simulink model "Control_try_final_2020b"  (R2020b)
settings: Solver=VariableStepAuto  StartTime=0.0  StopTime=inf  RelTol=1e-3
undefined symbols (not defined in the file or in its folder): DiscIntNeverNeededParam
libraries: mobileRoboticsLib x25
(part 1 of 7)
settings Model: Creator=its_ghani  LastModifiedBy=nitis
settings DebuggingCC: SFMachineParentedDataDiag=error  UnderSpecifiedDimensionMsg=warning

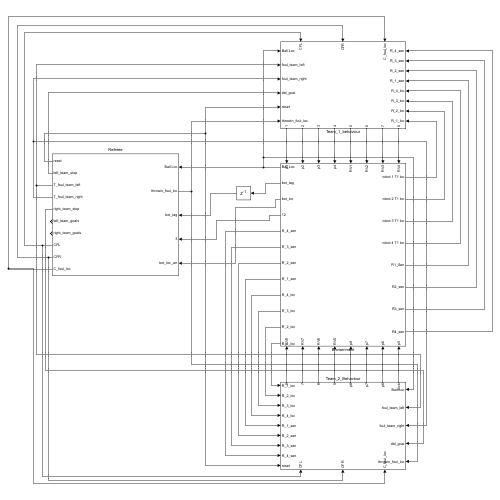
[thumbnail: Simulink's stored preview of the top-level diagram]
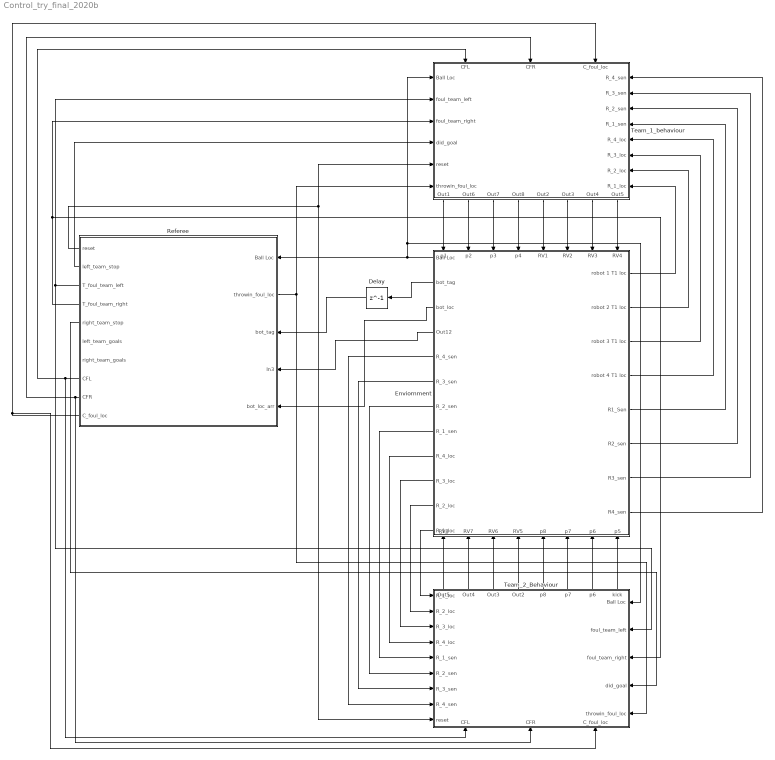
== system Control_try_final_2020b ==
  Delay : Delay  DelayLength=1
  Enviornment : Subsystem
      settings: PortSchema="{\"entries\":[{\"content\":{\"sides\":[{\"content\":{\"connectorIds\":[\"Out9\",\"Out10\",\"Out11\",\"Out12\",\"Out13\",\"Out14\",\"Out15\",\"Out16\",\"Out17\",\"Out18\",\"Out19\",\"Out20\"]},\"type\":\"ConnectorPlacement.EquallySpacedRectSide\",\"uuid\":\"bfc4f995-18bb-40a5-813e-439d500b4bf9\"},{\"content\":{\"connectorIds\":[\"Out1\",\"Out2\",\"Out3\",\"Out4\",\"Out5\",\"Out6\",\"Out7\",\"Out8\"],\"side\":\"RIGHT\"},\"type\":\"ConnectorPlacement.EquallySpacedRectSide\",\"uuid\":\"3fb6b8a6-16df-4a59-8ba5-6321e26d1fdd\"},{\"content\":{\"connectorIds\":[\"In1\",\"In2\",\"In3\",\"In4\",\"In5\",\"In6\",\"In7\",\"In8\"],\"side\":\"TOP\"},\"type\":\"ConnectorPlacement.EquallySpacedRectSide\",\"uuid\":\"a9e4cd1b-3afe-4395-99fa-15aef12a4070\"},{\"content\":{\"connectorIds\":[\"In9\",\"In10\",\"In11\",\"In12\",\"In13\",\"In14\",\"In15\",\"In16\"],\"side\":\"BOTTOM\"},\"type\":\"ConnectorPlacement.EquallySpacedRectSide\",\"uuid\":\"078de565-4bd1-4f1b-9c98-125152a73844\"}]},\"type\":\"ConnectorPlacement.EquallySpacedConnector\",\"uuid\":\"a6ca697e-fe67-43ac-b669-91f3e6c836c9\"}],\"packageUris\":[\"http://schema.mathworks.com/mf0/Connector/R2020b\"],\"version\":\"1.0\"}"
  Referee : Subsystem
      settings: PortSchema="{\"entries\":[{\"content\":{\"sides\":[{\"content\":{\"connectorIds\":[\"In1\",\"Out11\",\"In2\",\"In3\",\"In4\"]},\"type\":\"ConnectorPlacement.EquallySpacedRectSide\",\"uuid\":\"24b9e11e-cd74-4a0c-9d20-0512ace72e94\"},{\"content\":{\"connectorIds\":[\"Out1\",\"Out2\",\"Out3\",\"Out4\",\"Out5\",\"Out6\",\"Out7\",\"Out8\",\"Out9\",\"Out10\"],\"side\":\"RIGHT\"},\"type\":\"ConnectorPlacement.EquallySpacedRectSide\",\"uuid\":\"9dfe8633-4d3d-43ab-8a9b-a2838e7b041b\"},{\"content\":{\"connectorIds\":[],\"side\":\"TOP\"},\"type\":\"ConnectorPlacement.EquallySpacedRectSide\",\"uuid\":\"dd8f60d5-a719-4603-9445-e84921578fa6\"}]},\"type\":\"ConnectorPlacement.EquallySpacedConnector\",\"uuid\":\"54df3931-ee61-4f2f-89b6-33f93cd52d65\"}],\"packageUris\":[\"http://schema.mathworks.com/mf0/Connector/R2020b\"],\"version\":\"1.0\"}"
  Team_1_behaviour : Subsystem
      settings: PortSchema="{\"entries\":[{\"content\":{\"sides\":[{\"content\":{\"connectorIds\":[\"In1\",\"In2\",\"In3\",\"In4\",\"In5\",\"In6\"]},\"type\":\"ConnectorPlacement.EquallySpacedRectSide\",\"uuid\":\"3d238569-03e8-47ba-93af-d09e13fdb2d4\"},{\"content\":{\"connectorIds\":[\"In10\",\"In11\",\"In12\",\"In13\",\"In14\",\"In15\",\"In16\",\"In17\"],\"side\":\"RIGHT\"},\"type\":\"ConnectorPlacement.EquallySpacedRectSide\",\"uuid\":\"12d8afb4-4727-4f82-8566-507ab080c6de\"},{\"content\":{\"connectorIds\":[\"In7\",\"In8\",\"In9\"],\"side\":\"TOP\"},\"type\":\"ConnectorPlacement.EquallySpacedRectSide\",\"uuid\":\"c52fa7ec-51b7-43be-84ca-6ce417c012c7\"},{\"content\":{\"connectorIds\":[\"Out1\",\"Out2\",\"Out3\",\"Out4\",\"Out5\",\"Out6\",\"Out7\",\"Out8\"],\"side\":\"BOTTOM\"},\"type\":\"ConnectorPlacement.EquallySpacedRectSide\",\"uuid\":\"1ba4ac49-8e90-4b3f-8374-c14756940453\"}]},\"type\":\"ConnectorPlacement.EquallySpacedConnector\",\"uuid\":\"883bb5df-d6b2-498f-94a4-3b94e28c6a8f\"}],\"packageUris\":[\"http://schema.mathworks.com/mf0/Connector/R2020b\"],\"version\":\"1.0\"}"
  Team_2_Behaviour : Subsystem
      settings: PortSchema="{\"entries\":[{\"content\":{\"sides\":[{\"content\":{\"connectorIds\":[\"In1\",\"In2\",\"In3\",\"In4\",\"In5\"]},\"type\":\"ConnectorPlacement.EquallySpacedRectSide\",\"uuid\":\"3d238569-03e8-47ba-93af-d09e13fdb2d4\"},{\"content\":{\"connectorIds\":[\"In9\",\"In10\",\"In11\",\"In12\",\"In13\",\"In14\",\"In15\",\"In16\",\"In17\"],\"side\":\"RIGHT\"},\"type\":\"ConnectorPlacement.EquallySpacedRectSide\",\"uuid\":\"12d8afb4-4727-4f82-8566-507ab080c6de\"},{\"content\":{\"connectorIds\":[\"In6\",\"In7\",\"In8\"],\"side\":\"TOP\"},\"type\":\"ConnectorPlacement.EquallySpacedRectSide\",\"uuid\":\"c52fa7ec-51b7-43be-84ca-6ce417c012c7\"},{\"content\":{\"connectorIds\":[\"Out1\",\"Out2\",\"Out3\",\"Out4\",\"Out5\",\"Out6\",\"Out7\",\"Out8\"],\"side\":\"BOTTOM\"},\"type\":\"ConnectorPlacement.EquallySpacedRectSide\",\"uuid\":\"1ba4ac49-8e90-4b3f-8374-c14756940453\"}]},\"type\":\"ConnectorPlacement.EquallySpacedConnector\",\"uuid\":\"883bb5df-d6b2-498f-94a4-3b94e28c6a8f\"}],\"packageUris\":[\"http://schema.mathworks.com/mf0/Connector/R2020b\"],\"version\":\"1.0\"}"
  wires:
  Enviornment/9(Ball Loc) -> Team_1_behaviour/1(Ball Loc), Team_2_Behaviour/5(Ball Loc), Referee/1(Ball Loc)
  Team_1_behaviour/5(Out2) -> Enviornment/5(RV1)
  Team_1_behaviour/6(Out3) -> Enviornment/6(RV2)
  Team_1_behaviour/7(Out4) -> Enviornment/7(RV3)
  Team_1_behaviour/8(Out5) -> Enviornment/8(RV4)
  Enviornment/1(robot 1 T1 loc) -> Team_1_behaviour/17(R_1_loc)
  Enviornment/2(robot 2 T1 loc) -> Team_1_behaviour/16(R_2_loc)
  Enviornment/3(robot 3 T1 loc) -> Team_1_behaviour/15(R_3_loc)
  Enviornment/4(robot 4 T1 loc) -> Team_1_behaviour/14(R_4_loc)
  Enviornment/5(R1_Sen) -> Team_1_behaviour/13(R_1_sen)
  Enviornment/6(R2_sen) -> Team_1_behaviour/12(R_2_sen)
  Enviornment/7(R3_sen) -> Team_1_behaviour/11(R_3_sen)
  Enviornment/8(R4_sen) -> Team_1_behaviour/10(R_4_sen)
  Team_1_behaviour/2(Out6) -> Enviornment/2(p2)
  Team_1_behaviour/3(Out7) -> Enviornment/3(p3)
  Team_1_behaviour/4(Out8) -> Enviornment/4(p4)
  Enviornment/10(bot_tag) -> Delay/1
  Enviornment/11(bot_loc) -> Referee/4(bot_loc_arr)
  Team_2_Behaviour/1(kick) -> Enviornment/16(p5)
  Team_2_Behaviour/2(p6) -> Enviornment/15(p6)
  Team_2_Behaviour/3(p7) -> Enviornment/14(p7)
  Team_2_Behaviour/4(p8) -> Enviornment/13(p8)
  Team_2_Behaviour/5(Out2) -> Enviornment/12(RV5)
  Team_2_Behaviour/6(Out3) -> Enviornment/11(RV6)
  Team_2_Behaviour/7(Out4) -> Enviornment/10(RV7)
  Team_2_Behaviour/8(Out5) -> Enviornment/9(RV8)
  Enviornment/20(R_1_loc) -> Team_2_Behaviour/17(R_1_loc)
  Enviornment/19(R_2_loc) -> Team_2_Behaviour/16(R_2_loc)
  Enviornment/18(R_3_loc) -> Team_2_Behaviour/15(R_3_loc)
  Enviornment/17(R_4_loc) -> Team_2_Behaviour/14(R_4_loc)
  Enviornment/16(R_1_sen) -> Team_2_Behaviour/13(R_1_sen)
  Enviornment/15(R_2_sen) -> Team_2_Behaviour/12(R_2_sen)
  Enviornment/14(R_3_sen) -> Team_2_Behaviour/11(R_3_sen)
  Enviornment/13(R_4_sen) -> Team_2_Behaviour/10(R_4_sen)
  Team_1_behaviour/1(Out1) -> Enviornment/1(p1)
  Referee/1(reset) -> Team_1_behaviour/5(reset), Team_2_Behaviour/9(reset)
  Referee/2(left_team_stop) -> Team_1_behaviour/4(did_goal)
  Referee/5(right_team_stop) -> Team_2_Behaviour/2(did_goal)
  Referee/3(T_foul_team_left) -> Team_2_Behaviour/4(foul_team_left), Team_1_behaviour/2(foul_team_left)
  Referee/4(T_foul_team_right) -> Team_2_Behaviour/3(foul_team_right), Team_1_behaviour/3(foul_team_right)
  Referee/11(throwin_foul_loc) -> Team_2_Behaviour/1(throwin_foul_loc), Team_1_behaviour/6(throwin_foul_loc)
  Delay/1 -> Referee/2(bot_tag)
  Referee/8(CFL) -> Team_1_behaviour/7(CFL), Team_2_Behaviour/8(CFL)
  Referee/9(CFR) -> Team_1_behaviour/8(CFR), Team_2_Behaviour/7(CFR)
  Referee/10(C_foul_loc) -> Team_2_Behaviour/6(C_foul_loc), Team_1_behaviour/9(C_foul_loc)
  Enviornment/12(Out12) -> Referee/3(In3)

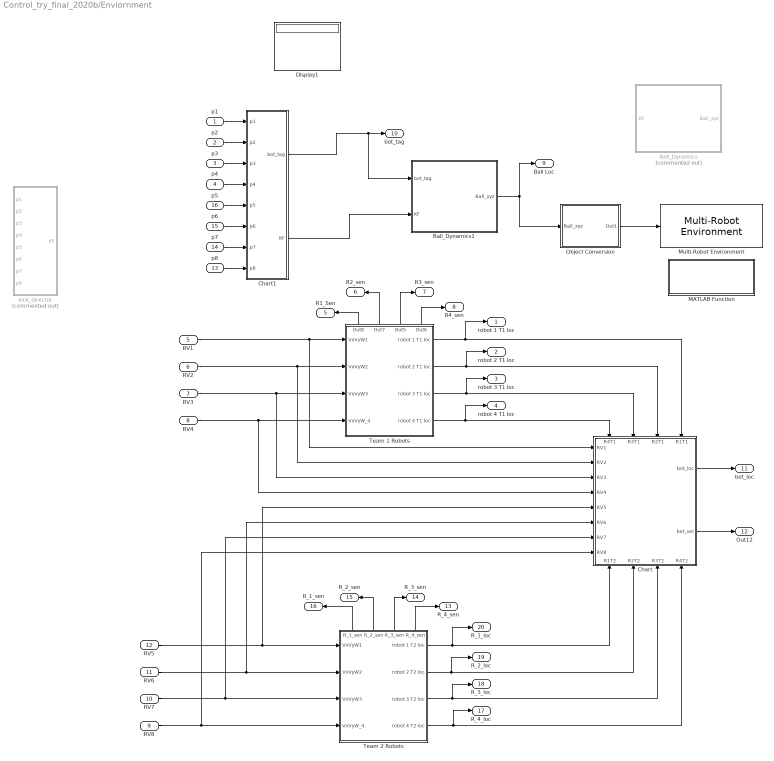
== system Control_try_final_2020b/Enviornment ==
  p1 : Inport  PortDimensions=4
  p2 : Inport  Port=2  PortDimensions=4
  p3 : Inport  Port=3  PortDimensions=4
  p4 : Inport  Port=4  PortDimensions=4
  RV1 : Inport  Port=5
  RV2 : Inport  Port=6
  RV3 : Inport  Port=7
  RV4 : Inport  Port=8
  RV8 : Inport  Port=9
  RV7 : Inport  Port=10
  RV6 : Inport  Port=11
  RV5 : Inport  Port=12
  p8 : Inport  Port=13  PortDimensions=4
  p7 : Inport  Port=14  PortDimensions=4
  p6 : Inport  Port=15  PortDimensions=4
  p5 : Inport  Port=16  PortDimensions=4
  "\tTeam 1 Robots" : Subsystem
      settings: PortSchema="{\"entries\":[{\"content\":{\"sides\":[{\"content\":{\"connectorIds\":[\"In1\",\"In2\",\"In3\",\"In4\"]},\"type\":\"ConnectorPlacement.EquallySpacedRectSide\",\"uuid\":\"e759642f-fbca-4f1e-b212-daca2c4962f8\"},{\"content\":{\"connectorIds\":[\"Out1\",\"Out2\",\"Out3\",\"Out4\"],\"side\":\"RIGHT\"},\"type\":\"ConnectorPlacement.EquallySpacedRectSide\",\"uuid\":\"6e1699fa-b246-4758-836f-1d4c98857b70\"},{\"content\":{\"connectorIds\":[\"Out5\",\"Out6\",\"Out7\",\"Out8\"],\"side\":\"TOP\"},\"type\":\"ConnectorPlacement.EquallySpacedRectSide\",\"uuid\":\"c1cf0a96-808a-4241-9d01-181cc4ce2a4d\"},{\"content\":{\"connectorIds\":[],\"side\":\"BOTTOM\"},\"type\":\"ConnectorPlacement.EquallySpacedRectSide\",\"uuid\":\"1a7f648f-16d5-4a09-b479-d6590fa53252\"}]},\"type\":\"ConnectorPlacement.EquallySpacedConnector\",\"uuid\":\"5972ed04-ecdd-4117-bf5d-456318b5c4b8\"}],\"packageUris\":[\"http://schema.mathworks.com/mf0/Connector/R2020b\"],\"version\":\"1.0\"}"
  "\tTeam 2 Robots" : Subsystem
      settings: PortSchema="{\"entries\":[{\"content\":{\"sides\":[{\"content\":{\"connectorIds\":[\"In1\",\"In2\",\"In3\",\"In4\"]},\"type\":\"ConnectorPlacement.EquallySpacedRectSide\",\"uuid\":\"e759642f-fbca-4f1e-b212-daca2c4962f8\"},{\"content\":{\"connectorIds\":[\"Out1\",\"Out2\",\"Out3\",\"Out4\"],\"side\":\"RIGHT\"},\"type\":\"ConnectorPlacement.EquallySpacedRectSide\",\"uuid\":\"6e1699fa-b246-4758-836f-1d4c98857b70\"},{\"content\":{\"connectorIds\":[\"Out5\",\"Out6\",\"Out7\",\"Out8\"],\"side\":\"TOP\"},\"type\":\"ConnectorPlacement.EquallySpacedRectSide\",\"uuid\":\"c1cf0a96-808a-4241-9d01-181cc4ce2a4d\"},{\"content\":{\"connectorIds\":[],\"side\":\"BOTTOM\"},\"type\":\"ConnectorPlacement.EquallySpacedRectSide\",\"uuid\":\"1a7f648f-16d5-4a09-b479-d6590fa53252\"}]},\"type\":\"ConnectorPlacement.EquallySpacedConnector\",\"uuid\":\"5972ed04-ecdd-4117-bf5d-456318b5c4b8\"}],\"packageUris\":[\"http://schema.mathworks.com/mf0/Connector/R2020b\"],\"version\":\"1.0\"}"
  Ball_Dynamics : Subsystem  Commented=on
  Ball_Dynamics1 : Subsystem
  Chart : Stateflow chart  TreatAsAtomicUnit=on
      settings: PortSchema="{\"entries\":[{\"content\":{\"sides\":[{\"content\":{\"connectorIds\":[\"In1\",\"In2\",\"In3\",\"In4\",\"In6\",\"In7\",\"In5\",\"In8\"]},\"type\":\"ConnectorPlacement.EquallySpacedRectSide\",\"uuid\":\"f94597f5-b931-46ba-a6a2-82ef940fcb13\"},{\"content\":{\"connectorIds\":[\"Out1\",\"Out2\"],\"side\":\"RIGHT\"},\"type\":\"ConnectorPlacement.EquallySpacedRectSide\",\"uuid\":\"0de80a09-1ed4-4b2b-aafe-6337a06ba998\"},{\"content\":{\"connectorIds\":[\"In13\",\"In14\",\"In15\",\"In16\"],\"side\":\"TOP\"},\"type\":\"ConnectorPlacement.EquallySpacedRectSide\",\"uuid\":\"f3cbd75f-0570-4224-b4a7-f582d3326f83\"},{\"content\":{\"connectorIds\":[\"In9\",\"In10\",\"In11\",\"In12\"],\"side\":\"BOTTOM\"},\"type\":\"ConnectorPlacement.EquallySpacedRectSide\",\"uuid\":\"407d67c2-1282-447f-b8c3-2ff3cae03a1f\"}]},\"type\":\"ConnectorPlacement.EquallySpacedConnector\",\"uuid\":\"17e3c346-79d8-441f-9c0c-3b96471ef7ab\"}],\"packageUris\":[\"http://schema.mathworks.com/mf0/Connector/R2020b\"],\"version\":\"1.0\"}"
  Chart1 : Stateflow chart  TreatAsAtomicUnit=on
  Display1 : Display
  MATLAB Function : MATLAB Function  TreatAsAtomicUnit=on
  Multi-Robot Environment : mobileRoboticsLib/Environments/Multi-Robot Environment  numRobots=8  showWaypoints=off  showObjects=on  objectColors=[1 0 0;0 1 0;0 0 1]  objectMarkers='c'  showRobotIds=on  plotSensorLines=on
      settings: SourceProductName=Mobile Robotics Simulation Toolbox
  Object Conversion : Subsystem
  kick_director : Subsystem  Commented=on
  robot 1 T1 loc : Outport
  robot 2 T1 loc : Outport  Port=2
  robot 3 T1 loc : Outport  Port=3
  robot 4 T1 loc : Outport  Port=4
  R1_Sen : Outport  Port=5
  R2_sen : Outport  Port=6
  R3_sen : Outport  Port=7
  R4_sen : Outport  Port=8
  Ball Loc : Outport  Port=9
  bot_tag : Outport  Port=10
  bot_loc : Outport  Port=11
  Out12 : Outport  Port=12
  R_4_sen : Outport  Port=13
  R_3_sen : Outport  Port=14
  R_2_sen : Outport  Port=15
  R_1_sen : Outport  Port=16
  R_4_loc : Outport  Port=17
  R_3_loc : Outport  Port=18
  R_2_loc : Outport  Port=19
  R_1_loc : Outport  Port=20
  wires:
  "\tTeam 1 Robots"/1(robot 1 T1 loc) -> robot 1 T1 loc/1, Chart/16(R1T1)
  Object Conversion/1(Out1) -> Multi-Robot Environment/1
  "\tTeam 1 Robots"/2(robot 2 T1 loc) -> robot 2 T1 loc/1, Chart/15(R2T1)
  "\tTeam 1 Robots"/3(robot 3 T1 loc) -> robot 3 T1 loc/1, Chart/14(R3T1)
  "\tTeam 1 Robots"/4(robot 4 T1 loc) -> robot 4 T1 loc/1, Chart/13(R4T1)
  RV1/1 -> Chart/1(RV1), "\tTeam 1 Robots"/1(VxVyW1)
  "\tTeam 1 Robots"/5(Out8) -> R1_Sen/1
  "\tTeam 1 Robots"/6(Out7) -> R2_sen/1
  "\tTeam 1 Robots"/7(Out5) -> R3_sen/1
  "\tTeam 1 Robots"/8(Out6) -> R4_sen/1
  "\tTeam 2 Robots"/4(robot 4 T2 loc) -> R_4_loc/1, Chart/12(R4T2)
  "\tTeam 2 Robots"/1(robot 1 T2 loc) -> R_1_loc/1, Chart/9(R1T2)
  "\tTeam 2 Robots"/2(robot 2 T2 loc) -> R_2_loc/1, Chart/10(R2T2)
  "\tTeam 2 Robots"/3(robot 3 T2 loc) -> R_3_loc/1, Chart/11(R3T2)
  Chart/1(bot_loc) -> bot_loc/1
  Ball_Dynamics1/1(Ball_xyz) -> Ball Loc/1, Object Conversion/1(Ball_xyz)
  RV5/1 -> Chart/6(RV5), "\tTeam 2 Robots"/1(VxVyW1)
  "\tTeam 2 Robots"/6(R_2_sen) -> R_2_sen/1
  "\tTeam 2 Robots"/7(R_3_sen) -> R_3_sen/1
  "\tTeam 2 Robots"/5(R_1_sen) -> R_1_sen/1
  "\tTeam 2 Robots"/8(R_4_sen) -> R_4_sen/1
  p1/1 -> Chart1/1(p1)
  p2/1 -> Chart1/2(p2)
  p3/1 -> Chart1/3(p3)
  p4/1 -> Chart1/4(p4)
  p5/1 -> Chart1/5(p5)
  p6/1 -> Chart1/6(p6)
  p7/1 -> Chart1/7(p7)
  p8/1 -> Chart1/8(p8)
  Chart1/2(KF) -> Ball_Dynamics1/2(KF)
  Chart1/1(bot_tag) -> Ball_Dynamics1/1(bot_tag), bot_tag/1
  RV8/1 -> Chart/8(RV8), "\tTeam 2 Robots"/4(VxVyW_4)
  RV2/1 -> Chart/2(RV2), "\tTeam 1 Robots"/2(VxVyW2)
  RV3/1 -> Chart/3(RV3), "\tTeam 1 Robots"/3(VxVyW3)
  RV4/1 -> Chart/4(RV4), "\tTeam 1 Robots"/4(VxVyW_4)
  RV6/1 -> Chart/7(RV6), "\tTeam 2 Robots"/2(VxVyW2)
  RV7/1 -> Chart/5(RV7), "\tTeam 2 Robots"/3(VxVyW3)
  Chart/2(bot_vel) -> Out12/1

== system Control_try_final_2020b/Referee ==
  Ball Loc : Inport
  bot_tag : Inport  Port=2
  In3 : Inport  Port=3
  bot_loc_arr : Inport  Port=4
  Chart : Stateflow chart  TreatAsAtomicUnit=on
  Corner : Stateflow chart  TreatAsAtomicUnit=on
  Demux : Demux  Outputs=3
  GOAL : Stateflow chart  TreatAsAtomicUnit=on
      settings: PortSchema="{\"entries\":[{\"content\":{\"sides\":[{\"content\":{\"connectorIds\":[\"In1\",\"In2\",\"In3\"]},\"type\":\"ConnectorPlacement.EquallySpacedRectSide\",\"uuid\":\"4d055f86-b6e4-40f8-8e5a-f88426a8f4c4\"},{\"content\":{\"connectorIds\":[\"Out1\",\"Out5\",\"Out3\",\"Out4\",\"Out2\"],\"side\":\"RIGHT\"},\"type\":\"ConnectorPlacement.EquallySpacedRectSide\",\"uuid\":\"6dafae19-6ec2-41d7-a60c-cff09e299cdb\"},{\"content\":{\"connectorIds\":[],\"side\":\"TOP\"},\"type\":\"ConnectorPlacement.EquallySpacedRectSide\",\"uuid\":\"9f5e82fb-41f6-4c76-b3de-1e77cfc54a18\"}]},\"type\":\"ConnectorPlacement.EquallySpacedConnector\",\"uuid\":\"d854df09-5db2-4850-aa8e-94906c2af310\"}],\"packageUris\":[\"http://schema.mathworks.com/mf0/Connector/R2020b\"],\"version\":\"1.0\"}"
  Throwing : Stateflow chart  TreatAsAtomicUnit=on
  reset : Outport
  left_team_stop : Outport  Port=2
  T_foul_team_left : Outport  Port=3
  T_foul_team_right : Outport  Port=4
  right_team_stop : Outport  Port=5
  left_team_goals : Outport  Port=6
  right_team_goals : Outport  Port=7
  CFL : Outport  Port=8
  CFR : Outport  Port=9
  C_foul_loc : Outport  Port=10
  throwin_foul_loc : Outport  Port=11
  wires:
  Ball Loc/1 -> Demux/1
  Demux/1 -> GOAL/1(X), Throwing/1(X), Corner/2(X)
  Demux/2 -> GOAL/2(Y), Throwing/3(Y), Corner/3(Y)
  Demux/3 -> GOAL/3(Z)
  GOAL/1(left_team_goal) -> left_team_goals/1
  GOAL/5(right_team_goal) -> right_team_goals/1
  GOAL/2(reset) -> reset/1
  bot_tag/1 -> Corner/1(ball_tag), Throwing/2(bot_tag)
  bot_loc_arr/1 -> Chart/2(bot_loc_arr)
  GOAL/4(right_team_stop) -> right_team_stop/1
  GOAL/3(left_team_stop) -> left_team_stop/1
  Throwing/2(foul_team_left) -> T_foul_team_left/1
  Throwing/1(foul_team_right) -> T_foul_team_right/1
  Throwing/3(throwin_foul_loc) -> throwin_foul_loc/1
  Corner/3(C_foul_loc) -> C_foul_loc/1
  Corner/2(CFL) -> CFL/1
  Corner/1(CFR) -> CFR/1
  In3/1 -> Chart/1(bot_vel)

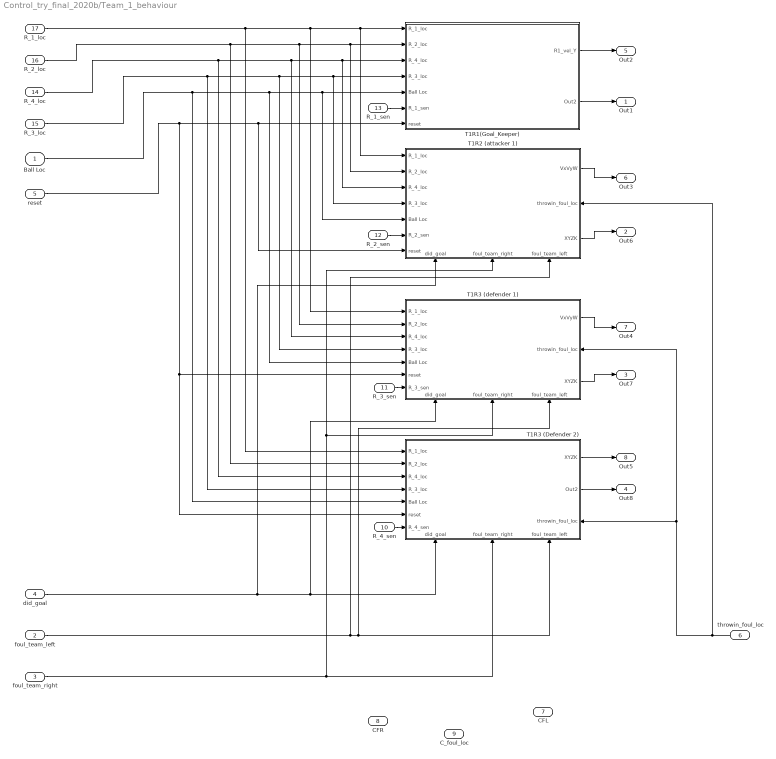
== system Control_try_final_2020b/Team_1_behaviour ==
  Ball Loc : Inport
  foul_team_left : Inport  Port=2
  foul_team_right : Inport  Port=3
  did_goal : Inport  Port=4
  reset : Inport  Port=5
  throwin_foul_loc : Inport  Port=6
  CFL : Inport  Port=7
  CFR : Inport  Port=8
  C_foul_loc : Inport  Port=9
  R_4_sen : Inport  Port=10
  R_3_sen : Inport  Port=11
  R_2_sen : Inport  Port=12
  R_1_sen : Inport  Port=13
  R_4_loc : Inport  Port=14
  R_3_loc : Inport  Port=15
  R_2_loc : Inport  Port=16
  R_1_loc : Inport  Port=17
  T1R1(Goal_Keeper) : Subsystem
  T1R2 (attacker 1) : Subsystem
      settings: PortSchema="{\"entries\":[{\"content\":{\"sides\":[{\"content\":{\"connectorIds\":[\"In1\",\"In2\",\"In3\",\"In4\",\"In5\",\"In6\",\"In7\"]},\"type\":\"ConnectorPlacement.EquallySpacedRectSide\",\"uuid\":\"970e53f5-0a77-471a-b839-4d72993ac113\"},{\"content\":{\"connectorIds\":[\"Out1\",\"In11\",\"Out2\"],\"side\":\"RIGHT\"},\"type\":\"ConnectorPlacement.EquallySpacedRectSide\",\"uuid\":\"b4f21133-1799-4814-963e-0f46ba79bd15\"},{\"content\":{\"connectorIds\":[],\"side\":\"TOP\"},\"type\":\"ConnectorPlacement.EquallySpacedRectSide\",\"uuid\":\"b11bbb03-05f4-411e-9610-26b6f9bf001d\"},{\"content\":{\"connectorIds\":[\"In8\",\"In9\",\"In10\"],\"side\":\"BOTTOM\"},\"type\":\"ConnectorPlacement.EquallySpacedRectSide\",\"uuid\":\"303a1a36-f5d7-4d15-b6f4-55568a48a6c3\"}]},\"type\":\"ConnectorPlacement.EquallySpacedConnector\",\"uuid\":\"9d40740d-7bec-4cd7-8121-739ec5dca381\"}],\"packageUris\":[\"http://schema.mathworks.com/mf0/Connector/R2020b\"],\"version\":\"1.0\"}"
  T1R3 (Defender 2) : Subsystem
      settings: PortSchema="{\"entries\":[{\"content\":{\"sides\":[{\"content\":{\"connectorIds\":[\"In1\",\"In2\",\"In3\",\"In4\",\"In5\",\"In6\",\"In7\"]},\"type\":\"ConnectorPlacement.EquallySpacedRectSide\",\"uuid\":\"970e53f5-0a77-471a-b839-4d72993ac113\"},{\"content\":{\"connectorIds\":[\"Out1\",\"Out2\",\"In11\"],\"side\":\"RIGHT\"},\"type\":\"ConnectorPlacement.EquallySpacedRectSide\",\"uuid\":\"b4f21133-1799-4814-963e-0f46ba79bd15\"},{\"content\":{\"connectorIds\":[],\"side\":\"TOP\"},\"type\":\"ConnectorPlacement.EquallySpacedRectSide\",\"uuid\":\"b11bbb03-05f4-411e-9610-26b6f9bf001d\"},{\"content\":{\"connectorIds\":[\"In8\",\"In9\",\"In10\"],\"side\":\"BOTTOM\"},\"type\":\"ConnectorPlacement.EquallySpacedRectSide\",\"uuid\":\"1ea9a003-1cbb-4940-9cbf-9a8dc4be1575\"}]},\"type\":\"ConnectorPlacement.EquallySpacedConnector\",\"uuid\":\"9d40740d-7bec-4cd7-8121-739ec5dca381\"}],\"packageUris\":[\"http://schema.mathworks.com/mf0/Connector/R2020b\"],\"version\":\"1.0\"}"
  T1R3 (defender 1) : Subsystem
      settings: PortSchema="{\"entries\":[{\"content\":{\"sides\":[{\"content\":{\"connectorIds\":[\"In1\",\"In2\",\"In3\",\"In4\",\"In5\",\"In6\",\"In7\"]},\"type\":\"ConnectorPlacement.EquallySpacedRectSide\",\"uuid\":\"970e53f5-0a77-471a-b839-4d72993ac113\"},{\"content\":{\"connectorIds\":[\"Out1\",\"In11\",\"Out2\"],\"side\":\"RIGHT\"},\"type\":\"ConnectorPlacement.EquallySpacedRectSide\",\"uuid\":\"b4f21133-1799-4814-963e-0f46ba79bd15\"},{\"content\":{\"connectorIds\":[],\"side\":\"TOP\"},\"type\":\"ConnectorPlacement.EquallySpacedRectSide\",\"uuid\":\"b11bbb03-05f4-411e-9610-26b6f9bf001d\"},{\"content\":{\"connectorIds\":[\"In8\",\"In9\",\"In10\"],\"side\":\"BOTTOM\"},\"type\":\"ConnectorPlacement.EquallySpacedRectSide\",\"uuid\":\"9d6502f6-0cb3-4e7b-b72a-712aec65b358\"}]},\"type\":\"ConnectorPlacement.EquallySpacedConnector\",\"uuid\":\"9d40740d-7bec-4cd7-8121-739ec5dca381\"}],\"packageUris\":[\"http://schema.mathworks.com/mf0/Connector/R2020b\"],\"version\":\"1.0\"}"
  Out1 : Outport
  Out6 : Outport  Port=2
  Out7 : Outport  Port=3
  Out8 : Outport  Port=4
  Out2 : Outport  Port=5
  Out3 : Outport  Port=6
  Out4 : Outport  Port=7
  Out5 : Outport  Port=8
  wires:
  T1R1(Goal_Keeper)/1(R1_vel_Y) -> Out2/1
  R_1_sen/1 -> T1R1(Goal_Keeper)/6(R_1_sen)
  R_1_loc/1 -> T1R3 (Defender 2)/1(R_1_loc), T1R3 (defender 1)/1(R_1_loc), T1R1(Goal_Keeper)/1(R_1_loc), T1R2 (attacker 1)/1(R_1_loc)
  R_2_loc/1 -> T1R3 (Defender 2)/2(R_2_loc), T1R3 (defender 1)/2(R_2_loc), T1R1(Goal_Keeper)/2(R_2_loc), T1R2 (attacker 1)/2(R_2_loc)
  R_4_loc/1 -> T1R3 (Defender 2)/3(R_4_loc), T1R3 (defender 1)/3(R_4_loc), T1R1(Goal_Keeper)/3(R_4_loc), T1R2 (attacker 1)/3(R_4_loc)
  R_3_loc/1 -> T1R3 (Defender 2)/4(R_3_loc), T1R3 (defender 1)/4(R_3_loc), T1R1(Goal_Keeper)/4(R_3_loc), T1R2 (attacker 1)/4(R_3_loc)
  Ball Loc/1 -> T1R3 (Defender 2)/5(Ball Loc), T1R3 (defender 1)/5(Ball Loc), T1R1(Goal_Keeper)/5(Ball Loc), T1R2 (attacker 1)/5(Ball Loc)
  R_2_sen/1 -> T1R2 (attacker 1)/6(R_2_sen)
  R_3_sen/1 -> T1R3 (defender 1)/7(R_3_sen)
  R_4_sen/1 -> T1R3 (Defender 2)/7(R_4_sen)
  T1R2 (attacker 1)/1(VxVyW) -> Out3/1
  T1R3 (defender 1)/1(VxVyW) -> Out4/1
  T1R3 (Defender 2)/1(XYZK) -> Out5/1
  T1R2 (attacker 1)/2(XYZK) -> Out6/1
  T1R3 (defender 1)/2(XYZK) -> Out7/1
  T1R3 (Defender 2)/2(Out2) -> Out8/1
  T1R1(Goal_Keeper)/2(Out2) -> Out1/1
  reset/1 -> T1R3 (defender 1)/6(reset), T1R3 (Defender 2)/6(reset), T1R1(Goal_Keeper)/7(reset), T1R2 (attacker 1)/7(reset)
  did_goal/1 -> T1R3 (Defender 2)/8(did_goal), T1R3 (defender 1)/8(did_goal), T1R2 (attacker 1)/8(did_goal)
  foul_team_left/1 -> T1R2 (attacker 1)/10(foul_team_left), T1R3 (defender 1)/10(foul_team_left), T1R3 (Defender 2)/10(foul_team_left)
  throwin_foul_loc/1 -> T1R2 (attacker 1)/11(throwin_foul_loc), T1R3 (defender 1)/11(throwin_foul_loc), T1R3 (Defender 2)/11(throwin_foul_loc)
  foul_team_right/1 -> T1R3 (defender 1)/9(foul_team_right), T1R2 (attacker 1)/9(foul_team_right), T1R3 (Defender 2)/9(foul_team_right)

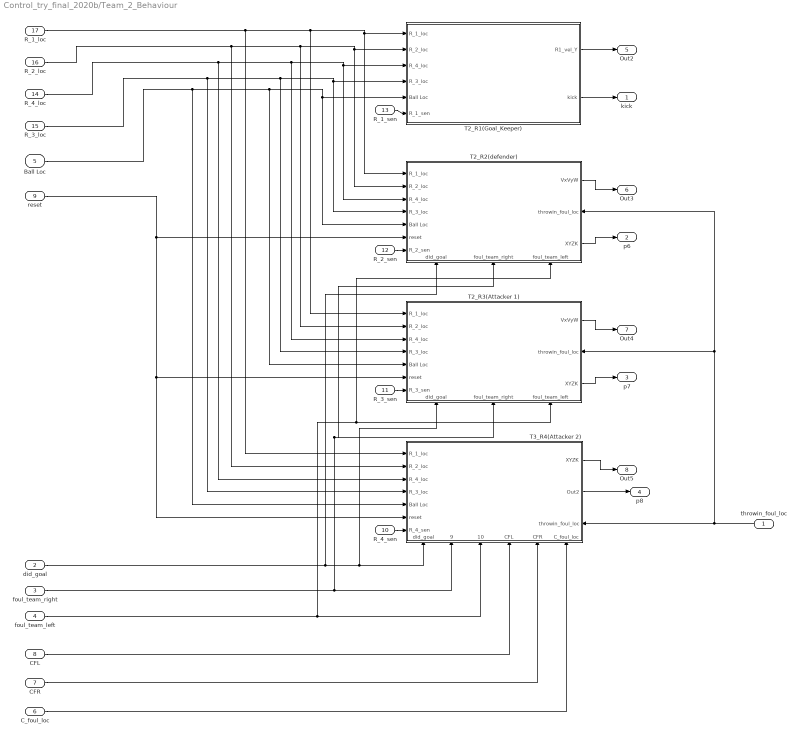
== system Control_try_final_2020b/Team_2_Behaviour ==
  throwin_foul_loc : Inport
  did_goal : Inport  Port=2
  foul_team_right : Inport  Port=3
  foul_team_left : Inport  Port=4
  Ball Loc : Inport  Port=5
  C_foul_loc : Inport  Port=6
  CFR : Inport  Port=7
  CFL : Inport  Port=8
  reset : Inport  Port=9
  R_4_sen : Inport  Port=10
  R_3_sen : Inport  Port=11
  R_2_sen : Inport  Port=12
  R_1_sen : Inport  Port=13
  R_4_loc : Inport  Port=14
  R_3_loc : Inport  Port=15
  R_2_loc : Inport  Port=16
  R_1_loc : Inport  Port=17
  T2_R1(Goal_Keeper) : Subsystem
  T2_R2(defender) : Subsystem
      settings: PortSchema="{\"entries\":[{\"content\":{\"sides\":[{\"content\":{\"connectorIds\":[\"In1\",\"In2\",\"In3\",\"In4\",\"In5\",\"In6\",\"In7\"]},\"type\":\"ConnectorPlacement.EquallySpacedRectSide\",\"uuid\":\"970e53f5-0a77-471a-b839-4d72993ac113\"},{\"content\":{\"connectorIds\":[\"Out1\",\"In11\",\"Out2\"],\"side\":\"RIGHT\"},\"type\":\"ConnectorPlacement.EquallySpacedRectSide\",\"uuid\":\"b4f21133-1799-4814-963e-0f46ba79bd15\"},{\"content\":{\"connectorIds\":[],\"side\":\"TOP\"},\"type\":\"ConnectorPlacement.EquallySpacedRectSide\",\"uuid\":\"b11bbb03-05f4-411e-9610-26b6f9bf001d\"},{\"content\":{\"connectorIds\":[\"In8\",\"In9\",\"In10\"],\"side\":\"BOTTOM\"},\"type\":\"ConnectorPlacement.EquallySpacedRectSide\",\"uuid\":\"e3d04837-b11c-4a80-91fc-07d9315080e1\"}]},\"type\":\"ConnectorPlacement.EquallySpacedConnector\",\"uuid\":\"9d40740d-7bec-4cd7-8121-739ec5dca381\"}],\"packageUris\":[\"http://schema.mathworks.com/mf0/Connector/R2020b\"],\"version\":\"1.0\"}"
  T2_R3(Attacker 1) : Subsystem
      settings: PortSchema="{\"entries\":[{\"content\":{\"sides\":[{\"content\":{\"connectorIds\":[\"In1\",\"In2\",\"In3\",\"In4\",\"In5\",\"In6\",\"In7\"]},\"type\":\"ConnectorPlacement.EquallySpacedRectSide\",\"uuid\":\"970e53f5-0a77-471a-b839-4d72993ac113\"},{\"content\":{\"connectorIds\":[\"Out1\",\"In11\",\"Out2\"],\"side\":\"RIGHT\"},\"type\":\"ConnectorPlacement.EquallySpacedRectSide\",\"uuid\":\"b4f21133-1799-4814-963e-0f46ba79bd15\"},{\"content\":{\"connectorIds\":[],\"side\":\"TOP\"},\"type\":\"ConnectorPlacement.EquallySpacedRectSide\",\"uuid\":\"b11bbb03-05f4-411e-9610-26b6f9bf001d\"},{\"content\":{\"connectorIds\":[\"In8\",\"In9\",\"In10\"],\"side\":\"BOTTOM\"},\"type\":\"ConnectorPlacement.EquallySpacedRectSide\",\"uuid\":\"51c3f414-bb29-49ed-bca1-9e09266b77a9\"}]},\"type\":\"ConnectorPlacement.EquallySpacedConnector\",\"uuid\":\"9d40740d-7bec-4cd7-8121-739ec5dca381\"}],\"packageUris\":[\"http://schema.mathworks.com/mf0/Connector/R2020b\"],\"version\":\"1.0\"}"
  T3_R4(Attacker 2) : Subsystem
      settings: PortSchema="{\"entries\":[{\"content\":{\"sides\":[{\"content\":{\"connectorIds\":[\"In1\",\"In2\",\"In3\",\"In4\",\"In5\",\"In6\",\"In7\"]},\"type\":\"ConnectorPlacement.EquallySpacedRectSide\",\"uuid\":\"970e53f5-0a77-471a-b839-4d72993ac113\"},{\"content\":{\"connectorIds\":[\"Out1\",\"Out2\",\"In14\"],\"side\":\"RIGHT\"},\"type\":\"ConnectorPlacement.EquallySpacedRectSide\",\"uuid\":\"b4f21133-1799-4814-963e-0f46ba79bd15\"},{\"content\":{\"connectorIds\":[],\"side\":\"TOP\"},\"type\":\"ConnectorPlacement.EquallySpacedRectSide\",\"uuid\":\"b11bbb03-05f4-411e-9610-26b6f9bf001d\"},{\"content\":{\"connectorIds\":[\"In8\",\"In9\",\"In10\",\"In11\",\"In12\",\"In13\"],\"side\":\"BOTTOM\"},\"type\":\"ConnectorPlacement.EquallySpacedRectSide\",\"uuid\":\"8ec21c7a-9592-41d9-bf7f-d73460ffbc72\"}]},\"type\":\"ConnectorPlacement.EquallySpacedConnector\",\"uuid\":\"9d40740d-7bec-4cd7-8121-739ec5dca381\"}],\"packageUris\":[\"http://schema.mathworks.com/mf0/Connector/R2020b\"],\"version\":\"1.0\"}"
  kick : Outport
  p6 : Outport  Port=2
  p7 : Outport  Port=3
  p8 : Outport  Port=4
  Out2 : Outport  Port=5
  Out3 : Outport  Port=6
  Out4 : Outport  Port=7
  Out5 : Outport  Port=8
  wires:
  T2_R1(Goal_Keeper)/1(R1_vel_Y) -> Out2/1
  R_1_sen/1 -> T2_R1(Goal_Keeper)/6(R_1_sen)
  R_1_loc/1 -> T3_R4(Attacker 2)/1(R_1_loc), T2_R3(Attacker 1)/1(R_1_loc), T2_R2(defender)/1(R_1_loc), T2_R1(Goal_Keeper)/1(R_1_loc)
  R_2_loc/1 -> T3_R4(Attacker 2)/2(R_2_loc), T2_R3(Attacker 1)/2(R_2_loc), T2_R2(defender)/2(R_2_loc), T2_R1(Goal_Keeper)/2(R_2_loc)
  R_4_loc/1 -> T3_R4(Attacker 2)/3(R_4_loc), T2_R3(Attacker 1)/3(R_4_loc), T2_R2(defender)/3(R_4_loc), T2_R1(Goal_Keeper)/3(R_4_loc)
  R_3_loc/1 -> T3_R4(Attacker 2)/4(R_3_loc), T2_R3(Attacker 1)/4(R_3_loc), T2_R2(defender)/4(R_3_loc), T2_R1(Goal_Keeper)/4(R_3_loc)
  Ball Loc/1 -> T3_R4(Attacker 2)/5(Ball Loc), T2_R3(Attacker 1)/5(Ball Loc), T2_R2(defender)/5(Ball Loc), T2_R1(Goal_Keeper)/5(Ball Loc)
  R_2_sen/1 -> T2_R2(defender)/7(R_2_sen)
  R_3_sen/1 -> T2_R3(Attacker 1)/7(R_3_sen)
  R_4_sen/1 -> T3_R4(Attacker 2)/7(R_4_sen)
  T2_R2(defender)/1(VxVyW) -> Out3/1
  T2_R3(Attacker 1)/1(VxVyW) -> Out4/1
  T3_R4(Attacker 2)/1(XYZK) -> Out5/1
  T2_R1(Goal_Keeper)/2(kick) -> kick/1
  T2_R2(defender)/2(XYZK) -> p6/1
  T2_R3(Attacker 1)/2(XYZK) -> p7/1
  T3_R4(Attacker 2)/2(Out2) -> p8/1
  reset/1 -> T3_R4(Attacker 2)/6(reset), T2_R3(Attacker 1)/6(reset), T2_R2(defender)/6(reset)
  did_goal/1 -> T2_R3(Attacker 1)/8(did_goal), T3_R4(Attacker 2)/8(did_goal), T2_R2(defender)/8(did_goal)
  throwin_foul_loc/1 -> T2_R3(Attacker 1)/11(throwin_foul_loc), T2_R2(defender)/11(throwin_foul_loc), T3_R4(Attacker 2)/14(throwin_foul_loc)
  foul_team_left/1 -> T2_R2(defender)/10(foul_team_left), T2_R3(Attacker 1)/10(foul_team_left), T3_R4(Attacker 2)/10(foul_team_left)
  foul_team_right/1 -> T2_R2(defender)/9(foul_team_right), T2_R3(Attacker 1)/9(foul_team_right), T3_R4(Attacker 2)/9(foul_team_right)
  CFL/1 -> T3_R4(Attacker 2)/11(CFL)
  CFR/1 -> T3_R4(Attacker 2)/12(CFR)
  C_foul_loc/1 -> T3_R4(Attacker 2)/13(C_foul_loc)

== system Control_try_final_2020b/Enviornment/	Team 1 Robots ==
  VxVyW1 : Inport
  VxVyW2 : Inport  Port=2
  VxVyW3 : Inport  Port=3
  VxVyW_4 : Inport  Port=4
  Goal_keeper : mobileRoboticsLib/Utilities/Generic Vehicle Simulation  initX=1.5  initY=4  initAngle=0  Ts=0.05
      settings: SourceProductName=Mobile Robotics Simulation Toolbox
  Robot 1 Vis : mobileRoboticsLib/Environments/Multi-Robot Visualizer  idx=1  radius=0.5  robotColor=[0 0 1]  showTraj=on  hasLidar=off  sensorOffset=[0,0]  scanAngles=[-pi/4, 0, pi/4]  hasObjDetector=off  objDetectorOffset=[0,0]  objDetectorAngle=0  objDetectorFOV=pi/3  objDetectorMaxRange=5
      settings: SourceProductName=Mobile Robotics Simulation Toolbox
  Robot 1 Vis1 : mobileRoboticsLib/Environments/Multi-Robot Visualizer  idx=2  radius=0.5  robotColor=[0 0 1]  showTraj=on  hasLidar=off  sensorOffset=[0,0]  scanAngles=[-pi/4, 0, pi/4]  hasObjDetector=off  objDetectorOffset=[0,0]  objDetectorAngle=0  objDetectorFOV=pi/3  objDetectorMaxRange=5
      settings: SourceProductName=Mobile Robotics Simulation Toolbox
  Robot 1 Vis2 : mobileRoboticsLib/Environments/Multi-Robot Visualizer  idx=3  radius=0.5  robotColor=[0 0 1]  showTraj=on  hasLidar=off  sensorOffset=[0,0]  scanAngles=[-pi/4, 0, pi/4]  hasObjDetector=off  objDetectorOffset=[0,0]  objDetectorAngle=0  objDetectorFOV=pi/3  objDetectorMaxRange=5
      settings: SourceProductName=Mobile Robotics Simulation Toolbox
  Robot 1 Vis3 : mobileRoboticsLib/Environments/Multi-Robot Visualizer  idx=4  radius=0.5  robotColor=[0 0 1]  showTraj=on  hasLidar=off  sensorOffset=[0,0]  scanAngles=[-pi/4, 0, pi/4]  hasObjDetector=off  objDetectorOffset=[0,0]  objDetectorAngle=0  objDetectorFOV=pi/3  objDetectorMaxRange=5
      settings: SourceProductName=Mobile Robotics Simulation Toolbox
  Robot 2 : mobileRoboticsLib/Utilities/Generic Vehicle Simulation  initX=3.25  initY=2.5  initAngle=0  Ts=0.05
      settings: SourceProductName=Mobile Robotics Simulation Toolbox
  Robot 3 : mobileRoboticsLib/Utilities/Generic Vehicle Simulation  initX=3.25  initY=5.5  initAngle=0  Ts=0.05
      settings: SourceProductName=Mobile Robotics Simulation Toolbox
  Robot 4 : mobileRoboticsLib/Utilities/Generic Vehicle Simulation  initX=5  initY=3  initAngle=0  Ts=0.05
      settings: SourceProductName=Mobile Robotics Simulation Toolbox
  Robot Detector : mobileRoboticsLib/Environments/Robot Detector  robotIdx=1  sensorOffset=[ 0, 0 ]  sensorAngle=0  fieldOfView=pi/3  maxRange=3  maxDetections=7  sampleTime=0.1
      settings: SourceProductName=Mobile Robotics Simulation Toolbox
  Robot Detector1 : mobileRoboticsLib/Environments/Robot Detector  robotIdx=3  sensorOffset=[ 0, 0 ]  sensorAngle=0  fieldOfView=pi/3  maxRange=1.5  maxDetections=7  sampleTime=0.1
      settings: SourceProductName=Mobile Robotics Simulation Toolbox
  Robot Detector2 : mobileRoboticsLib/Environments/Robot Detector  robotIdx=4  sensorOffset=[ 0, 0 ]  sensorAngle=0  fieldOfView=pi/3  maxRange=1.5  maxDetections=7  sampleTime=0.1
      settings: SourceProductName=Mobile Robotics Simulation Toolbox
  Robot Detector3 : mobileRoboticsLib/Environments/Robot Detector  robotIdx=2  sensorOffset=[ 0, 0 ]  sensorAngle=0  fieldOfView=pi/3  maxRange=1.5  maxDetections=7  sampleTime=0.1
      settings: SourceProductName=Mobile Robotics Simulation Toolbox
  robot 1 T1 loc : Outport
  robot 2 T1 loc : Outport  Port=2
  robot 3 T1 loc : Outport  Port=3
  robot 4 T1 loc : Outport  Port=4
  Out8 : Outport  Port=5
  Out7 : Outport  Port=6
  Out5 : Outport  Port=7
  Out6 : Outport  Port=8
  wires:
  Goal_keeper/1 -> robot 1 T1 loc/1, Robot 1 Vis/1
  VxVyW1/1 -> Goal_keeper/1
  VxVyW2/1 -> Robot 2/1
  Robot 2/1 -> robot 2 T1 loc/1, Robot 1 Vis1/1
  Robot 3/1 -> Robot 1 Vis2/1, robot 3 T1 loc/1
  VxVyW3/1 -> Robot 3/1
  VxVyW_4/1 -> Robot 4/1
  Robot 4/1 -> robot 4 T1 loc/1, Robot 1 Vis3/1
  Robot Detector3/1 -> Out7/1
  Robot Detector1/1 -> Out5/1
  Robot Detector2/1 -> Out6/1
  Robot Detector/1 -> Out8/1

== system Control_try_final_2020b/Enviornment/	Team 2 Robots ==
  VxVyW1 : Inport
  VxVyW2 : Inport  Port=2
  VxVyW3 : Inport  Port=3
  VxVyW_4 : Inport  Port=4
  Goal_keeper : mobileRoboticsLib/Utilities/Generic Vehicle Simulation  initX=9.5  initY=4  initAngle=pi  Ts=0.05
      settings: SourceProductName=Mobile Robotics Simulation Toolbox
  Robot 1 Vis : mobileRoboticsLib/Environments/Multi-Robot Visualizer  idx=5  radius=0.5  robotColor=[1 0 0]  showTraj=on  hasLidar=off  sensorOffset=[0,0]  scanAngles=[-pi/4, 0, pi/4]  hasObjDetector=off  objDetectorOffset=[0,0]  objDetectorAngle=0  objDetectorFOV=pi/3  objDetectorMaxRange=5
      settings: SourceProductName=Mobile Robotics Simulation Toolbox
  Robot 1 Vis1 : mobileRoboticsLib/Environments/Multi-Robot Visualizer  idx=6  radius=0.5  robotColor=[0.1 1 1]  showTraj=on  hasLidar=off  sensorOffset=[0,0]  scanAngles=[-pi/4, 0, pi/4]  hasObjDetector=off  objDetectorOffset=[0,0]  objDetectorAngle=0  objDetectorFOV=pi/3  objDetectorMaxRange=5
      settings: SourceProductName=Mobile Robotics Simulation Toolbox
  Robot 1 Vis2 : mobileRoboticsLib/Environments/Multi-Robot Visualizer  idx=7  radius=0.5  robotColor=[0 1 1]  showTraj=on  hasLidar=off  sensorOffset=[0,0]  scanAngles=[-pi/4, 0, pi/4]  hasObjDetector=off  objDetectorOffset=[0,0]  objDetectorAngle=0  objDetectorFOV=pi/3  objDetectorMaxRange=5
      settings: SourceProductName=Mobile Robotics Simulation Toolbox
  Robot 1 Vis3 : mobileRoboticsLib/Environments/Multi-Robot Visualizer  idx=8  radius=0.5  robotColor=[0 1 1]  showTraj=on  hasLidar=off  sensorOffset=[0,0]  scanAngles=[-pi/4, 0, pi/4]  hasObjDetector=off  objDetectorOffset=[0,0]  objDetectorAngle=0  objDetectorFOV=pi/3  objDetectorMaxRange=5
      settings: SourceProductName=Mobile Robotics Simulation Toolbox
  Robot 2 : mobileRoboticsLib/Utilities/Generic Vehicle Simulation  initX=7.25  initY=2.5  initAngle=pi  Ts=0.05
      settings: SourceProductName=Mobile Robotics Simulation Toolbox
  Robot 3 : mobileRoboticsLib/Utilities/Generic Vehicle Simulation  initX=7.5  initY=5.5  initAngle=pi  Ts=0.05
      settings: SourceProductName=Mobile Robotics Simulation Toolbox
  Robot 4 : mobileRoboticsLib/Utilities/Generic Vehicle Simulation  initX=6  initY=4  initAngle=pi  Ts=0.05
      settings: SourceProductName=Mobile Robotics Simulation Toolbox
  Robot Detector : mobileRoboticsLib/Environments/Robot Detector  robotIdx=5  sensorOffset=[ 0, 0 ]  sensorAngle=0  fieldOfView=pi/3  maxRange=1.5  maxDetections=7  sampleTime=0.1
      settings: SourceProductName=Mobile Robotics Simulation Toolbox
  Robot Detector1 : mobileRoboticsLib/Environments/Robot Detector  robotIdx=7  sensorOffset=[ 0, 0 ]  sensorAngle=0  fieldOfView=pi/3  maxRange=1.5  maxDetections=7  sampleTime=0.1
      settings: SourceProductName=Mobile Robotics Simulation Toolbox
  Robot Detector2 : mobileRoboticsLib/Environments/Robot Detector  robotIdx=8  sensorOffset=[ 0, 0 ]  sensorAngle=0  fieldOfView=pi/3  maxRange=1.5  maxDetections=7  sampleTime=0.1
      settings: SourceProductName=Mobile Robotics Simulation Toolbox
  Robot Detector3 : mobileRoboticsLib/Environments/Robot Detector  robotIdx=6  sensorOffset=[ 0, 0 ]  sensorAngle=0  fieldOfView=pi/3  maxRange=1.5  maxDetections=7  sampleTime=0.1
      settings: SourceProductName=Mobile Robotics Simulation Toolbox
  robot 1 T2 loc : Outport
  robot 2 T2 loc : Outport  Port=2
  robot 3 T2 loc : Outport  Port=3
  robot 4 T2 loc : Outport  Port=4
  R_1_sen : Outport  Port=5
  R_2_sen : Outport  Port=6
  R_3_sen : Outport  Port=7
  R_4_sen : Outport  Port=8
  wires:
  Goal_keeper/1 -> robot 1 T2 loc/1, Robot 1 Vis/1
  VxVyW1/1 -> Goal_keeper/1
  VxVyW2/1 -> Robot 2/1
  Robot 2/1 -> robot 2 T2 loc/1, Robot 1 Vis1/1
  Robot 3/1 -> Robot 1 Vis2/1, robot 3 T2 loc/1
  VxVyW3/1 -> Robot 3/1
  VxVyW_4/1 -> Robot 4/1
  Robot 4/1 -> robot 4 T2 loc/1, Robot 1 Vis3/1
  Robot Detector3/1 -> R_2_sen/1
  Robot Detector1/1 -> R_3_sen/1
  Robot Detector2/1 -> R_4_sen/1
  Robot Detector/1 -> R_1_sen/1

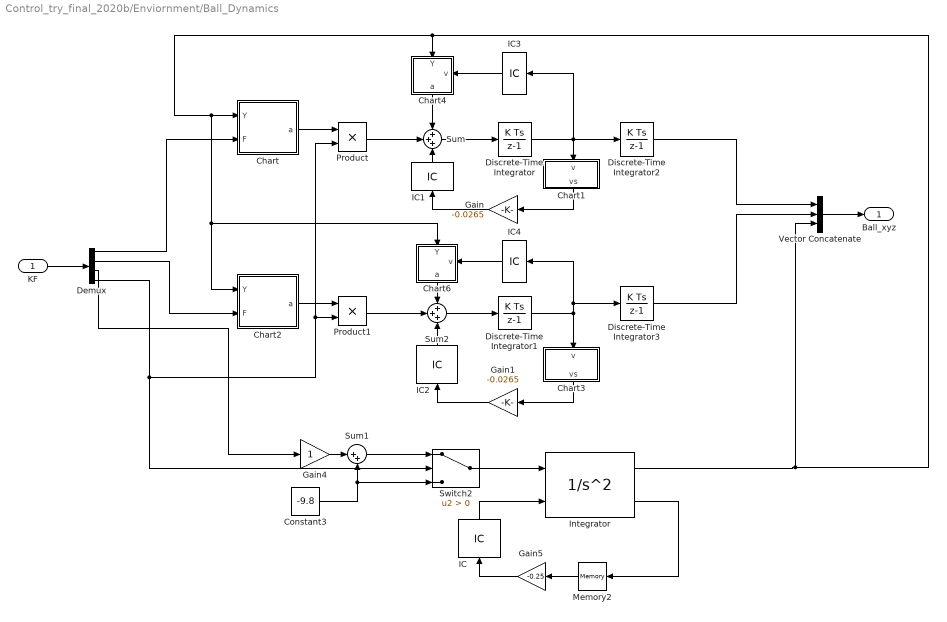
== system Control_try_final_2020b/Enviornment/Ball_Dynamics ==
  KF : Inport
  Chart : Stateflow chart  TreatAsAtomicUnit=on
  Chart1 : Stateflow chart  TreatAsAtomicUnit=on
      settings: PortSchema="{\"entries\":[{\"content\":{\"sides\":[{\"content\":{\"connectorIds\":[]},\"type\":\"ConnectorPlacement.EquallySpacedRectSide\",\"uuid\":\"edcb69b6-c92b-474e-86d7-1e52c2e82b28\"},{\"content\":{\"connectorIds\":[],\"side\":\"RIGHT\"},\"type\":\"ConnectorPlacement.EquallySpacedRectSide\",\"uuid\":\"df9771e4-6870-4305-9c84-3f71fcb76e6b\"},{\"content\":{\"connectorIds\":[\"In1\"],\"side\":\"TOP\"},\"type\":\"ConnectorPlacement.EquallySpacedRectSide\",\"uuid\":\"56b80241-156d-4669-9174-884a577f2013\"},{\"content\":{\"connectorIds\":[\"Out1\"],\"side\":\"BOTTOM\"},\"type\":\"ConnectorPlacement.EquallySpacedRectSide\",\"uuid\":\"179af6a7-cab5-4faa-a562-268e2d2e4d3e\"}]},\"type\":\"ConnectorPlacement.EquallySpacedConnector\",\"uuid\":\"707001f1-02b8-4f5e-ba3f-f155c99072e5\"}],\"packageUris\":[\"http://schema.mathworks.com/mf0/Connector/R2020b\"],\"version\":\"1.0\"}"
  Chart2 : Stateflow chart  TreatAsAtomicUnit=on
  Chart3 : Stateflow chart  TreatAsAtomicUnit=on
      settings: PortSchema="{\"entries\":[{\"content\":{\"sides\":[{\"content\":{\"connectorIds\":[]},\"type\":\"ConnectorPlacement.EquallySpacedRectSide\",\"uuid\":\"edcb69b6-c92b-474e-86d7-1e52c2e82b28\"},{\"content\":{\"connectorIds\":[],\"side\":\"RIGHT\"},\"type\":\"ConnectorPlacement.EquallySpacedRectSide\",\"uuid\":\"df9771e4-6870-4305-9c84-3f71fcb76e6b\"},{\"content\":{\"connectorIds\":[\"In1\"],\"side\":\"TOP\"},\"type\":\"ConnectorPlacement.EquallySpacedRectSide\",\"uuid\":\"56b80241-156d-4669-9174-884a577f2013\"},{\"content\":{\"connectorIds\":[\"Out1\"],\"side\":\"BOTTOM\"},\"type\":\"ConnectorPlacement.EquallySpacedRectSide\",\"uuid\":\"179af6a7-cab5-4faa-a562-268e2d2e4d3e\"}]},\"type\":\"ConnectorPlacement.EquallySpacedConnector\",\"uuid\":\"707001f1-02b8-4f5e-ba3f-f155c99072e5\"}],\"packageUris\":[\"http://schema.mathworks.com/mf0/Connector/R2020b\"],\"version\":\"1.0\"}"
  Chart4 : Stateflow chart  TreatAsAtomicUnit=on
      settings: PortSchema="{\"entries\":[{\"content\":{\"sides\":[{\"content\":{\"connectorIds\":[]},\"type\":\"ConnectorPlacement.EquallySpacedRectSide\",\"uuid\":\"edcb69b6-c92b-474e-86d7-1e52c2e82b28\"},{\"content\":{\"connectorIds\":[\"In2\"],\"side\":\"RIGHT\"},\"type\":\"ConnectorPlacement.EquallySpacedRectSide\",\"uuid\":\"df9771e4-6870-4305-9c84-3f71fcb76e6b\"},{\"content\":{\"connectorIds\":[\"In1\"],\"side\":\"TOP\"},\"type\":\"ConnectorPlacement.EquallySpacedRectSide\",\"uuid\":\"56b80241-156d-4669-9174-884a577f2013\"},{\"content\":{\"connectorIds\":[\"Out1\"],\"side\":\"BOTTOM\"},\"type\":\"ConnectorPlacement.EquallySpacedRectSide\",\"uuid\":\"6d9abc99-74e1-40c2-a49f-e0d9410a29cc\"}]},\"type\":\"ConnectorPlacement.EquallySpacedConnector\",\"uuid\":\"707001f1-02b8-4f5e-ba3f-f155c99072e5\"}],\"packageUris\":[\"http://schema.mathworks.com/mf0/Connector/R2020b\"],\"version\":\"1.0\"}"
  Chart6 : Stateflow chart  TreatAsAtomicUnit=on
      settings: PortSchema="{\"entries\":[{\"content\":{\"sides\":[{\"content\":{\"connectorIds\":[]},\"type\":\"ConnectorPlacement.EquallySpacedRectSide\",\"uuid\":\"edcb69b6-c92b-474e-86d7-1e52c2e82b28\"},{\"content\":{\"connectorIds\":[\"In2\"],\"side\":\"RIGHT\"},\"type\":\"ConnectorPlacement.EquallySpacedRectSide\",\"uuid\":\"df9771e4-6870-4305-9c84-3f71fcb76e6b\"},{\"content\":{\"connectorIds\":[\"In1\"],\"side\":\"TOP\"},\"type\":\"ConnectorPlacement.EquallySpacedRectSide\",\"uuid\":\"56b80241-156d-4669-9174-884a577f2013\"},{\"content\":{\"connectorIds\":[\"Out1\"],\"side\":\"BOTTOM\"},\"type\":\"ConnectorPlacement.EquallySpacedRectSide\",\"uuid\":\"6d9abc99-74e1-40c2-a49f-e0d9410a29cc\"}]},\"type\":\"ConnectorPlacement.EquallySpacedConnector\",\"uuid\":\"707001f1-02b8-4f5e-ba3f-f155c99072e5\"}],\"packageUris\":[\"http://schema.mathworks.com/mf0/Connector/R2020b\"],\"version\":\"1.0\"}"
  Constant3 : Constant  Value=-9.8
  Demux : Demux
  Discrete-Time Integrator : DiscreteIntegrator  SampleTime=-1  ICPrevOutput=DiscIntNeverNeededParam  ICPrevScaledInput=DiscIntNeverNeededParam
  Discrete-Time Integrator1 : DiscreteIntegrator  SampleTime=-1  ICPrevOutput=DiscIntNeverNeededParam  ICPrevScaledInput=DiscIntNeverNeededParam
  Discrete-Time Integrator2 : DiscreteIntegrator  InitialCondition=6.9  SampleTime=-1  ICPrevOutput=DiscIntNeverNeededParam  ICPrevScaledInput=DiscIntNeverNeededParam
  Discrete-Time Integrator3 : DiscreteIntegrator  InitialCondition=6.9  SampleTime=-1  ICPrevOutput=DiscIntNeverNeededParam  ICPrevScaledInput=DiscIntNeverNeededParam
  Gain : Gain  Gain=-0.0265
  Gain1 : Gain  Gain=-0.0265
  Gain4 : Gain
  Gain5 : Gain  Gain=-0.25
  IC : InitialCondition
  IC{1..4} (4 alike) : InitialCondition  Value=0
  Integrator : SecondOrderIntegrator  ICX=0  LimitX=on  LowerLimitX=0.0  StateNameX='Position'  ICSourceDXDT=external  StateNameDXDT='Velocity'  ReinitDXDTwhenXreachesSaturation=on
  Memory2 : Memory
  Product : Product
  Product1 : Product
  Sum : Sum  Inputs=+++
  Sum1 : Sum  Inputs=|++
  Sum2 : Sum  Inputs=+++
  Switch2 : Switch  Criteria=u2 > Threshold
  Vector Concatenate : Concatenate  NumInputs=3
  Ball_xyz : Outport
  wires:
  Constant3/1 -> Sum1/2, Switch2/3
  Integrator/2 -> Memory2/1
  Memory2/1 -> Gain5/1
  IC/1 -> Integrator/2
  Switch2/1 -> Integrator/1
  Sum1/1 -> Switch2/1
  Gain4/1 -> Sum1/1
  Demux/3 -> Gain4/1
  Demux/4 -> Switch2/2, Product/2, Product1/2
  Gain5/1 -> IC/1
  KF/1 -> Demux/1
  Gain/1 -> IC1/1
  Chart/1(a) -> Product/1
  Sum/1 -> Discrete-Time Integrator/1
  Discrete-Time Integrator1/1 -> IC4/1, Discrete-Time Integrator3/1, Chart3/1(v)
  Chart2/1(a) -> Product1/1
  Gain1/1 -> IC2/1
  Product1/1 -> Sum2/2
  Sum2/1 -> Discrete-Time Integrator1/1
  Demux/1 -> Chart/2(F)
  Demux/2 -> Chart2/2(F)
  Integrator/1 -> Vector Concatenate/3, Chart6/1(Y), Chart2/1(Y), Chart/1(Y), Chart4/1(Y)
  Chart1/1(vs) -> Gain/1
  Chart3/1(vs) -> Gain1/1
  IC3/1 -> Chart4/2(v)
  Discrete-Time Integrator/1 -> IC3/1, Discrete-Time Integrator2/1, Chart1/1(v)
  Product/1 -> Sum/2
  IC2/1 -> Sum2/3
  IC1/1 -> Sum/3
  IC4/1 -> Chart6/2(v)
  Chart4/1(a) -> Sum/1
  Chart6/1(a) -> Sum2/1
  Vector Concatenate/1 -> Ball_xyz/1
  Discrete-Time Integrator2/1 -> Vector Concatenate/1
  Discrete-Time Integrator3/1 -> Vector Concatenate/2

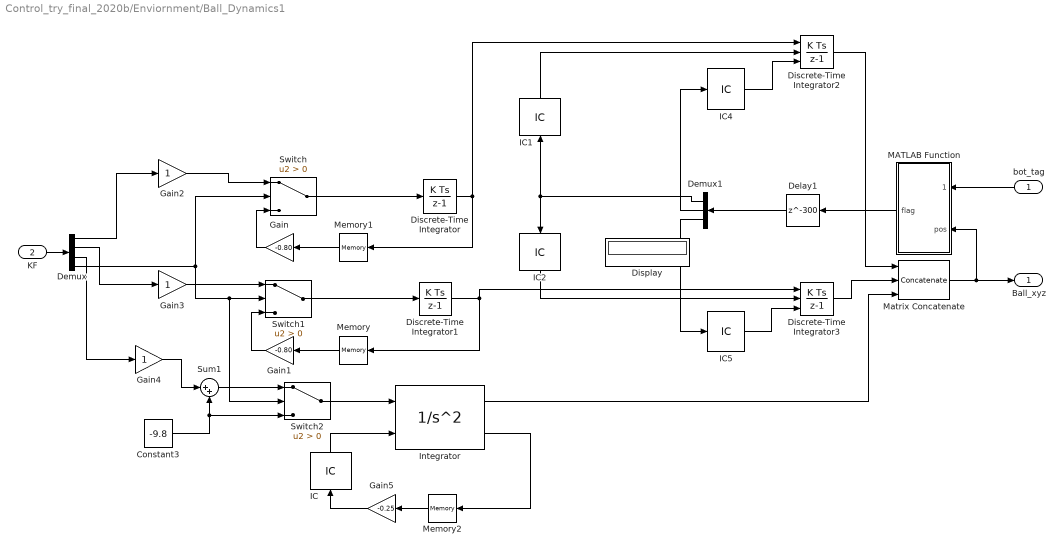
== system Control_try_final_2020b/Enviornment/Ball_Dynamics1 ==
  bot_tag : Inport
  KF : Inport  Port=2
  Constant3 : Constant  Value=-9.8
  Delay1 : Delay  DelayLength=300
  Demux : Demux
  Demux1 : Demux  Outputs=3
  Discrete-Time Integrator : DiscreteIntegrator  SampleTime=-1  ICPrevOutput=DiscIntNeverNeededParam  ICPrevScaledInput=DiscIntNeverNeededParam
  Discrete-Time Integrator1 : DiscreteIntegrator  SampleTime=-1  ICPrevOutput=DiscIntNeverNeededParam  ICPrevScaledInput=DiscIntNeverNeededParam
  Discrete-Time Integrator2 : DiscreteIntegrator  ExternalReset=rising  InitialConditionSource=external  InitialCondition=6  SampleTime=-1  ICPrevOutput=DiscIntNeverNeededParam  ICPrevScaledInput=DiscIntNeverNeededParam
  Discrete-Time Integrator3 : DiscreteIntegrator  ExternalReset=rising  InitialConditionSource=external  InitialCondition=6.9  SampleTime=-1  ICPrevOutput=DiscIntNeverNeededParam  ICPrevScaledInput=DiscIntNeverNeededParam
  Display : Display
  Gain : Gain  Gain=-0.80
  Gain1 : Gain  Gain=-0.80
  Gain2 : Gain
  Gain3 : Gain
  Gain4 : Gain
  Gain5 : Gain  Gain=-0.25
  IC : InitialCondition
  IC1 : InitialCondition  Value=0
  IC2 : InitialCondition  Value=0
  IC4 : InitialCondition  Value=5.5
  IC5 : InitialCondition  Value=4
  Integrator : SecondOrderIntegrator  ICX=0  LimitX=on  LowerLimitX=0.0  StateNameX='Position'  ICSourceDXDT=external  StateNameDXDT='Velocity'  ReinitDXDTwhenXreachesSaturation=on
  MATLAB Function : MATLAB Function  TreatAsAtomicUnit=on
  Matrix Concatenate : Concatenate  NumInputs=3  Mode=Multidimensional array  ConcatenateDimension=2
  Memory : Memory
  Memory1 : Memory
  Memory2 : Memory
  Sum1 : Sum  Inputs=|++
  Switch : Switch  Criteria=u2 > Threshold
  Switch1 : Switch  Criteria=u2 > Threshold
  Switch2 : Switch  Criteria=u2 > Threshold
  Ball_xyz : Outport
  wires:
  Gain/1 -> Switch/3
  Gain1/1 -> Switch1/3
  Discrete-Time Integrator/1 -> Memory1/1, Discrete-Time Integrator2/1
  Discrete-Time Integrator1/1 -> Memory/1, Discrete-Time Integrator3/1
  Gain2/1 -> Switch/1
  Gain3/1 -> Switch1/1
  Discrete-Time Integrator3/1 -> Matrix Concatenate/2
  Discrete-Time Integrator2/1 -> Matrix Concatenate/1
  Constant3/1 -> Sum1/2, Switch2/3
  Integrator/2 -> Memory2/1
  Memory2/1 -> Gain5/1
  IC/1 -> Integrator/2
  Switch2/1 -> Integrator/1
  Sum1/1 -> Switch2/1
  Gain4/1 -> Sum1/1
  Demux/1 -> Gain2/1
  Demux/2 -> Gain3/1
  Demux/3 -> Gain4/1
  Demux/4 -> Switch/2, Switch1/2, Switch2/2
  Gain5/1 -> IC/1
  KF/1 -> Demux/1
  IC1/1 -> Discrete-Time Integrator2/2
  IC2/1 -> Discrete-Time Integrator3/2
  Memory1/1 -> Gain/1
  Switch/1 -> Discrete-Time Integrator/1
  Memory/1 -> Gain1/1
  Switch1/1 -> Discrete-Time Integrator1/1
  Integrator/1 -> Matrix Concatenate/3
  Matrix Concatenate/1 -> MATLAB Function/2(pos), Ball_xyz/1
  IC5/1 -> Discrete-Time Integrator3/3
  IC4/1 -> Discrete-Time Integrator2/3
  MATLAB Function/1(flag) -> Delay1/1
  Demux1/2 -> IC4/1
  Demux1/3 -> IC5/1
  Demux1/1 -> IC1/1, IC2/1
  Delay1/1 -> Demux1/1
  bot_tag/1 -> MATLAB Function/1(bot_tag)

== system Control_try_final_2020b/Enviornment/Object Conversion ==
  Ball_xyz : Inport
  Ball : Constant
  Demux : Demux  Outputs=3
  Matrix Concatenate : Concatenate  NumInputs=3  Mode=Multidimensional array  ConcatenateDimension=2
  Out1 : Outport
  wires:
  Ball/1 -> Matrix Concatenate/3
  Matrix Concatenate/1 -> Out1/1
  Ball_xyz/1 -> Demux/1
  Demux/1 -> Matrix Concatenate/1
  Demux/2 -> Matrix Concatenate/2

== system Control_try_final_2020b/Enviornment/kick_director ==
  p1 : Inport
  p2 : Inport  Port=2
  p3 : Inport  Port=3
  p4 : Inport  Port=4
  p5 : Inport  Port=5
  p6 : Inport  Port=6
  p7 : Inport  Port=7
  p8 : Inport  Port=8
  Chart : Stateflow chart  TreatAsAtomicUnit=on
  KF : Outport
  wires:
  Chart/1(KF) -> KF/1
  p2/1 -> Chart/2(p2)
  p3/1 -> Chart/3(p3)
  p4/1 -> Chart/4(p4)
  p5/1 -> Chart/5(p5)
  p6/1 -> Chart/6(p6)
  p7/1 -> Chart/7(p7)
  p8/1 -> Chart/8(p8)
  p1/1 -> Chart/1(p1)

== system Control_try_final_2020b/Team_1_behaviour/T1R1(Goal_Keeper) ==
  R_1_loc : Inport
  R_2_loc : Inport  Port=2
  R_4_loc : Inport  Port=3
  R_3_loc : Inport  Port=4
  Ball Loc : Inport  Port=5
  R_1_sen : Inport  Port=6
  reset : Inport  Port=7
  Ball_in_D : Subsystem
      settings: PortSchema="{\"entries\":[{\"content\":{\"sides\":[{\"content\":{\"connectorIds\":[\"Out1\",\"Out2\"]},\"type\":\"ConnectorPlacement.EquallySpacedRectSide\",\"uuid\":\"be901545-21b9-45e5-bac5-a8cb9027aef5\"},{\"content\":{\"connectorIds\":[\"In1\",\"In2\",\"In3\"],\"side\":\"RIGHT\"},\"type\":\"ConnectorPlacement.EquallySpacedRectSide\",\"uuid\":\"b7c1eb84-2f14-4c7f-a74c-d56efbe0743e\"},{\"content\":{\"connectorIds\":[],\"side\":\"TOP\"},\"type\":\"ConnectorPlacement.EquallySpacedRectSide\",\"uuid\":\"aca41723-ed3f-4bd2-8fc1-457d075e3460\"}]},\"type\":\"ConnectorPlacement.EquallySpacedConnector\",\"uuid\":\"e10e22f1-c8f0-4dfc-85d2-4ba01528372d\"}],\"packageUris\":[\"http://schema.mathworks.com/mf0/Connector/R2020b\"],\"version\":\"1.0\"}"
  Chart : Stateflow chart  TreatAsAtomicUnit=on
  Demux : Demux  Outputs=3
  ball_out_of_D : Subsystem
  min_Distance_Finder : Subsystem
      settings: PortSchema="{\"entries\":[{\"content\":{\"sides\":[{\"content\":{\"connectorIds\":[\"In1\",\"In2\"]},\"type\":\"ConnectorPlacement.EquallySpacedRectSide\",\"uuid\":\"45cf91c7-7d38-4a19-bf35-d1d31095287a\"},{\"content\":{\"connectorIds\":[\"Out1\"],\"side\":\"RIGHT\"},\"type\":\"ConnectorPlacement.EquallySpacedRectSide\",\"uuid\":\"645394ba-2e5d-4060-b61c-cc9330ee0038\"},{\"content\":{\"connectorIds\":[\"In3\",\"In4\",\"In5\"],\"side\":\"TOP\"},\"type\":\"ConnectorPlacement.EquallySpacedRectSide\",\"uuid\":\"4fc56b73-04ec-476f-b487-f0e593f708ad\"},{\"content\":{\"connectorIds\":[],\"side\":\"BOTTOM\"},\"type\":\"ConnectorPlacement.EquallySpacedRectSide\",\"uuid\":\"cd306436-fd63-4e79-88e6-7a63c0840ed7\"}]},\"type\":\"ConnectorPlacement.EquallySpacedConnector\",\"uuid\":\"5cf2ee04-00eb-490b-958c-5fb90b43d325\"}],\"packageUris\":[\"http://schema.mathworks.com/mf0/Connector/R2020b\"],\"version\":\"1.0\"}"
  R1_vel_Y : Outport
  Out2 : Outport  Port=2
  wires:
  R_2_loc/1 -> min_Distance_Finder/3(R_2_loc)
  R_3_loc/1 -> min_Distance_Finder/4(R_3_loc)
  R_4_loc/1 -> min_Distance_Finder/5(R_4_loc)
  R_1_sen/1 -> min_Distance_Finder/1(R_1_sen)
  R_1_loc/1 -> min_Distance_Finder/2(R_1_loc), Ball_in_D/2(Robot 1 T1 Loc), ball_out_of_D/2(R_1_loc)
  min_Distance_Finder/1(kick_direction) -> Ball_in_D/3(In1), ball_out_of_D/1(kick_direction)
  Ball Loc/1 -> Demux/1, ball_out_of_D/3(Ball Loc), Ball_in_D/1(Ball Loc)
  Demux/1 -> Chart/1(X)
  Demux/2 -> Chart/2(Y)
  ball_out_of_D/1(Out2) -> Out2/1
  ball_out_of_D/2(R1_vel_Y) -> R1_vel_Y/1
